simulink model "TST_APP_DD1"  (R2016b)
settings: Solver=FixedStepDiscrete  StartTime=0.0  StopTime=simTime  FixedStep=sampleTime  RelTol=1e-3
values from neighbouring files (symbols this model uses):
  testCase = 1    [initTST_APP_DD1_001.m]    (also in initTST_APP_DD1_002.m = 2)
libraries: simulink x3
settings Model: Creator=wolf072601  LastModifiedBy=wolf072601
settings DebuggingCC: SignalRangeChecking=error

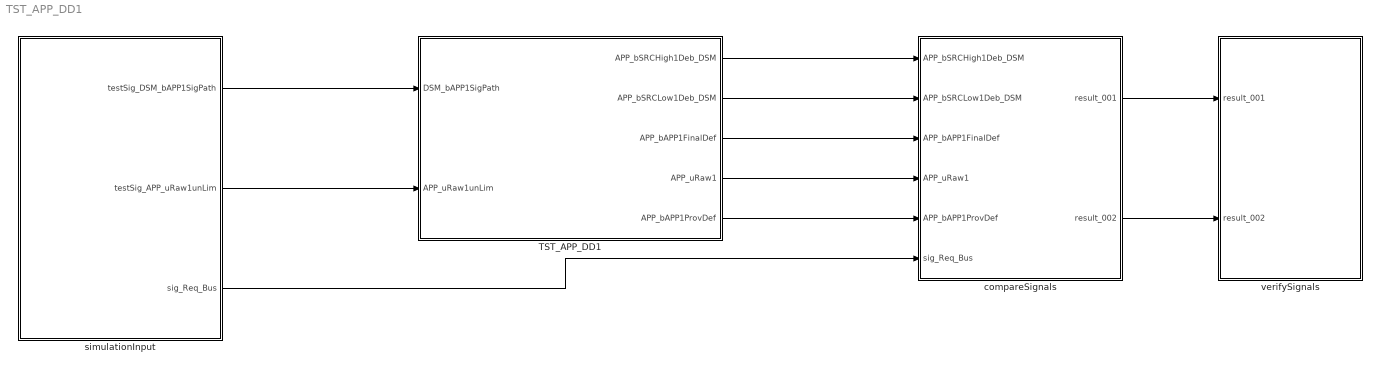
== system TST_APP_DD1 ==
  TST_APP_DD1 : Subsystem
  compareSignals : Subsystem
  simulationInput : Subsystem
  verifySignals : Subsystem
  wires:
  simulationInput/1(testSig_DSM_bAPP1SigPath) -> TST_APP_DD1/1(DSM_bAPP1SigPath)
  simulationInput/2(testSig_APP_uRaw1unLim) -> TST_APP_DD1/2(APP_uRaw1unLim)
  TST_APP_DD1/1(APP_bSRCHigh1Deb_DSM) -> compareSignals/1(APP_bSRCHigh1Deb_DSM)
  TST_APP_DD1/2(APP_bSRCLow1Deb_DSM) -> compareSignals/2(APP_bSRCLow1Deb_DSM)
  TST_APP_DD1/3(APP_bAPP1FinalDef) -> compareSignals/3(APP_bAPP1FinalDef)
  TST_APP_DD1/4(APP_uRaw1) -> compareSignals/4(APP_uRaw1)
  TST_APP_DD1/5(APP_bAPP1ProvDef) -> compareSignals/5(APP_bAPP1ProvDef)
  simulationInput/3(sig_Req_Bus) -> compareSignals/6(sig_Req_Bus)
  compareSignals/1(result_001) -> verifySignals/1(result_001)
  compareSignals/2(result_002) -> verifySignals/2(result_002)

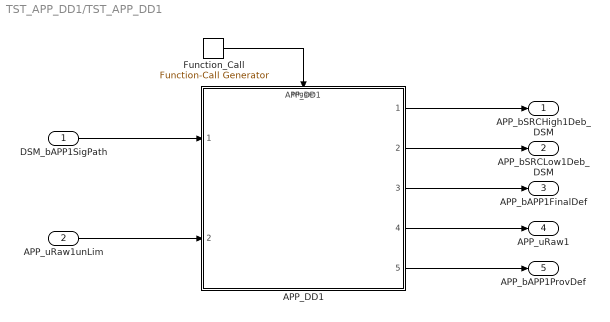
== system TST_APP_DD1/TST_APP_DD1 ==
  DSM_bAPP1SigPath : Inport
  APP_uRaw1unLim : Inport  Port=2
  APP_DD1 : ModelReference  ModelNameDialog=APP_DD1  SimulationMode=Normal  ModelReferenceVersion=1.21  TriggerPortName=function  TriggerPortTriggerType=function-call  TriggerPortStatesWhenEnabling=held
  Function_Call : simulink/Ports & Subsystems/Function-Call Generator  sample_time=sampleTime  numberOfIterations=1
  APP_bSRCHigh1Deb_DSM : Outport
  APP_bSRCLow1Deb_DSM : Outport  Port=2
  APP_bAPP1FinalDef : Outport  Port=3
  APP_uRaw1 : Outport  Port=4
  APP_bAPP1ProvDef : Outport  Port=5
  wires:
  Function_Call/1 -> APP_DD1/Trigger
  DSM_bAPP1SigPath/1 -> APP_DD1/1
  APP_uRaw1unLim/1 -> APP_DD1/2
  APP_DD1/1 -> APP_bSRCHigh1Deb_DSM/1
  APP_DD1/2 -> APP_bSRCLow1Deb_DSM/1
  APP_DD1/3 -> APP_bAPP1FinalDef/1
  APP_DD1/4 -> APP_uRaw1/1
  APP_DD1/5 -> APP_bAPP1ProvDef/1

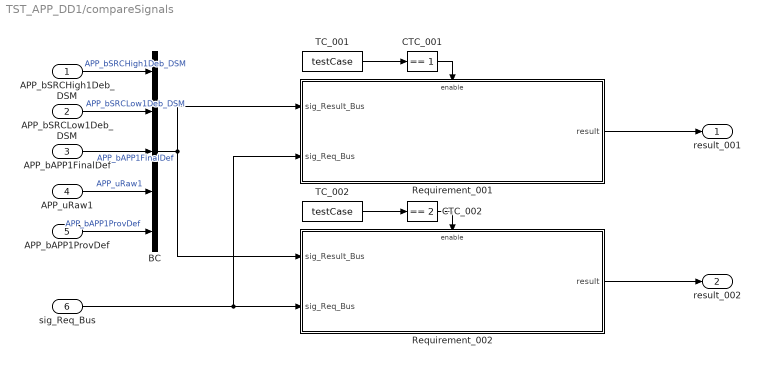
== system TST_APP_DD1/compareSignals ==
  APP_bSRCHigh1Deb_DSM : Inport
  APP_bSRCLow1Deb_DSM : Inport  Port=2
  APP_bAPP1FinalDef : Inport  Port=3
  APP_uRaw1 : Inport  Port=4
  APP_bAPP1ProvDef : Inport  Port=5
  sig_Req_Bus : Inport  Port=6
  BC : BusCreator  Inputs=5
  CTC_001 : simulink/Logic and Bit Operations/Compare To Constant  relop===  const=1  OutDataTypeStr=boolean
  CTC_002 : simulink/Logic and Bit Operations/Compare To Constant  relop===  const=2  OutDataTypeStr=boolean
  Requirement_001 : Subsystem
  Requirement_002 : Subsystem
  TC_001 : Constant  Value=testCase
  TC_002 : Constant  Value=testCase
  result_001 : Outport
  result_002 : Outport  Port=2
  wires:
  APP_bSRCHigh1Deb_DSM/1 -> BC/1  "APP_bSRCHigh1Deb_DSM"
  APP_bSRCLow1Deb_DSM/1 -> BC/2  "APP_bSRCLow1Deb_DSM"
  APP_bAPP1FinalDef/1 -> BC/3  "APP_bAPP1FinalDef"
  APP_uRaw1/1 -> BC/4  "APP_uRaw1"
  APP_bAPP1ProvDef/1 -> BC/5  "APP_bAPP1ProvDef"
  TC_001/1 -> CTC_001/1
  CTC_001/1 -> Requirement_001/Enable
  sig_Req_Bus/1 -> Requirement_002/2(sig_Req_Bus), Requirement_001/2(sig_Req_Bus)
  BC/1 -> Requirement_002/1(sig_Result_Bus), Requirement_001/1(sig_Result_Bus)
  Requirement_001/1(result) -> result_001/1
  TC_002/1 -> CTC_002/1
  CTC_002/1 -> Requirement_002/Enable
  Requirement_002/1(result) -> result_002/1

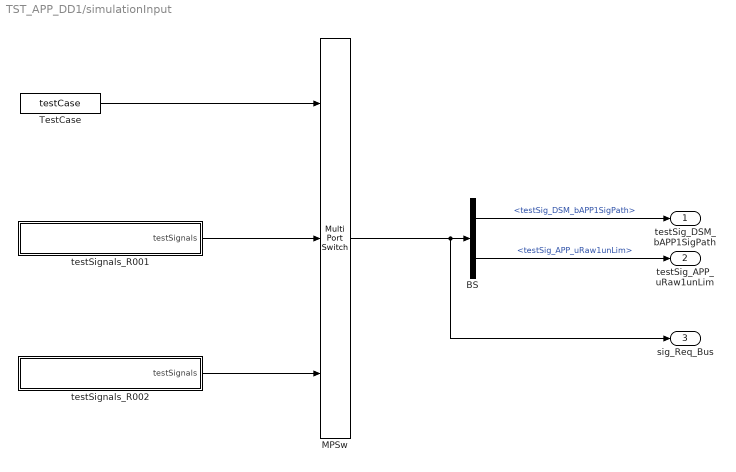
== system TST_APP_DD1/simulationInput ==
  BS : BusSelector  OutputSignals=testSig_DSM_bAPP1SigPath,testSig_APP_uRaw1unLim
  MPSw : MultiPortSwitch  Inputs=2  SaturateOnIntegerOverflow=on  InputSameDT=on
  TestCase : Constant  Value=testCase
  testSignals_R001 : Subsystem
  testSignals_R002 : Subsystem
  testSig_DSM_bAPP1SigPath : Outport
  testSig_APP_uRaw1unLim : Outport  Port=2
  sig_Req_Bus : Outport  Port=3
  wires:
  BS/1 -> testSig_DSM_bAPP1SigPath/1  "<testSig_DSM_bAPP1SigPath>"
  BS/2 -> testSig_APP_uRaw1unLim/1  "<testSig_APP_uRaw1unLim>"
  MPSw/1 -> BS/1, sig_Req_Bus/1
  TestCase/1 -> MPSw/1
  testSignals_R001/1(testSignals) -> MPSw/2
  testSignals_R002/1(testSignals) -> MPSw/3

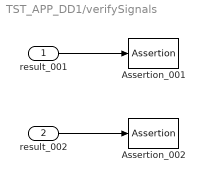
== system TST_APP_DD1/verifySignals ==
  result_001 : Inport
  result_002 : Inport  Port=2
  Assertion_001 : Assertion  Enabled=off
  Assertion_002 : Assertion
  wires:
  result_001/1 -> Assertion_001/1
  result_002/1 -> Assertion_002/1

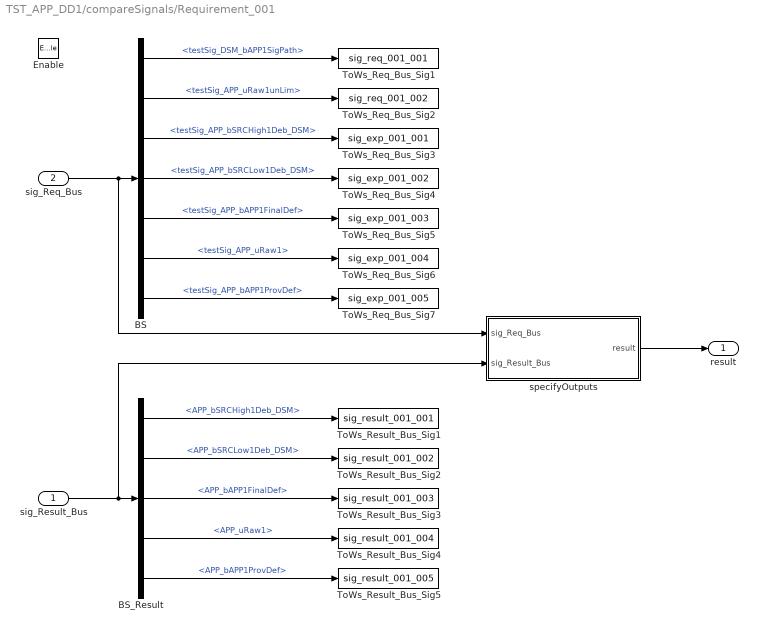
== system TST_APP_DD1/compareSignals/Requirement_001 ==
  sig_Result_Bus : Inport
  sig_Req_Bus : Inport  Port=2
  Enable : EnablePort
  BS : BusSelector  OutputSignals=testSig_DSM_bAPP1SigPath,testSig_APP_uRaw1unLim,testSig_APP_bSRCHigh1Deb_DSM,testSig_APP_bSRCLow1Deb_DSM,testSig_APP_bAPP1FinalDef,testSig_APP_uRaw1,testSig_APP_bAPP1ProvDef
  BS_Result : BusSelector  OutputSignals=APP_bSRCHigh1Deb_DSM,APP_bSRCLow1Deb_DSM,APP_bAPP1FinalDef,APP_uRaw1,APP_bAPP1ProvDef
  ToWs_Req_Bus_Sig1 : ToWorkspace  VariableName=sig_req_001_001  SaveFormat=Structure With Time
  ToWs_Req_Bus_Sig2 : ToWorkspace  VariableName=sig_req_001_002  SaveFormat=Structure With Time
  ToWs_Req_Bus_Sig3 : ToWorkspace  VariableName=sig_exp_001_001  SaveFormat=Structure With Time
  ToWs_Req_Bus_Sig4 : ToWorkspace  VariableName=sig_exp_001_002  SaveFormat=Structure With Time
  ToWs_Req_Bus_Sig5 : ToWorkspace  VariableName=sig_exp_001_003  SaveFormat=Structure With Time
  ToWs_Req_Bus_Sig6 : ToWorkspace  VariableName=sig_exp_001_004  SaveFormat=Structure With Time
  ToWs_Req_Bus_Sig7 : ToWorkspace  VariableName=sig_exp_001_005  SaveFormat=Structure With Time
  ToWs_Result_Bus_Sig1 : ToWorkspace  VariableName=sig_result_001_001  SaveFormat=Structure With Time
  ToWs_Result_Bus_Sig2 : ToWorkspace  VariableName=sig_result_001_002  SaveFormat=Structure With Time
  ToWs_Result_Bus_Sig3 : ToWorkspace  VariableName=sig_result_001_003  SaveFormat=Structure With Time
  ToWs_Result_Bus_Sig4 : ToWorkspace  VariableName=sig_result_001_004  SaveFormat=Structure With Time
  ToWs_Result_Bus_Sig5 : ToWorkspace  VariableName=sig_result_001_005  SaveFormat=Structure With Time
  specifyOutputs : Subsystem
  result : Outport
  wires:
  sig_Req_Bus/1 -> BS/1, specifyOutputs/1(sig_Req_Bus)
  BS/1 -> ToWs_Req_Bus_Sig1/1  "<testSig_DSM_bAPP1SigPath>"
  BS/2 -> ToWs_Req_Bus_Sig2/1  "<testSig_APP_uRaw1unLim>"
  BS/3 -> ToWs_Req_Bus_Sig3/1  "<testSig_APP_bSRCHigh1Deb_DSM>"
  BS/4 -> ToWs_Req_Bus_Sig4/1  "<testSig_APP_bSRCLow1Deb_DSM>"
  BS/5 -> ToWs_Req_Bus_Sig5/1  "<testSig_APP_bAPP1FinalDef>"
  BS/6 -> ToWs_Req_Bus_Sig6/1  "<testSig_APP_uRaw1>"
  BS/7 -> ToWs_Req_Bus_Sig7/1  "<testSig_APP_bAPP1ProvDef>"
  sig_Result_Bus/1 -> BS_Result/1, specifyOutputs/2(sig_Result_Bus)
  BS_Result/1 -> ToWs_Result_Bus_Sig1/1  "<APP_bSRCHigh1Deb_DSM>"
  BS_Result/2 -> ToWs_Result_Bus_Sig2/1  "<APP_bSRCLow1Deb_DSM>"
  BS_Result/3 -> ToWs_Result_Bus_Sig3/1  "<APP_bAPP1FinalDef>"
  BS_Result/4 -> ToWs_Result_Bus_Sig4/1  "<APP_uRaw1>"
  BS_Result/5 -> ToWs_Result_Bus_Sig5/1  "<APP_bAPP1ProvDef>"
  specifyOutputs/1(result) -> result/1

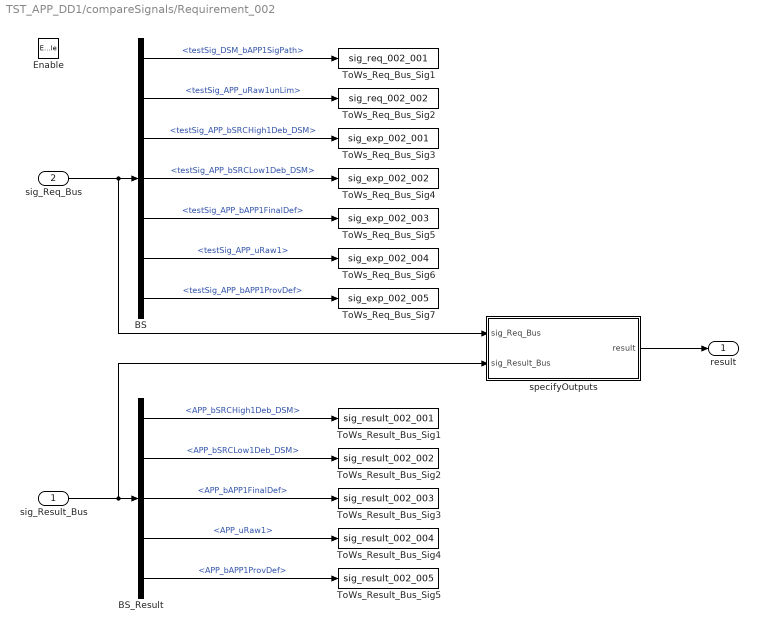
== system TST_APP_DD1/compareSignals/Requirement_002 ==
  sig_Result_Bus : Inport
  sig_Req_Bus : Inport  Port=2
  Enable : EnablePort
  BS : BusSelector  OutputSignals=testSig_DSM_bAPP1SigPath,testSig_APP_uRaw1unLim,testSig_APP_bSRCHigh1Deb_DSM,testSig_APP_bSRCLow1Deb_DSM,testSig_APP_bAPP1FinalDef,testSig_APP_uRaw1,testSig_APP_bAPP1ProvDef
  BS_Result : BusSelector  OutputSignals=APP_bSRCHigh1Deb_DSM,APP_bSRCLow1Deb_DSM,APP_bAPP1FinalDef,APP_uRaw1,APP_bAPP1ProvDef
  ToWs_Req_Bus_Sig1 : ToWorkspace  VariableName=sig_req_002_001  SaveFormat=Structure With Time
  ToWs_Req_Bus_Sig2 : ToWorkspace  VariableName=sig_req_002_002  SaveFormat=Structure With Time
  ToWs_Req_Bus_Sig3 : ToWorkspace  VariableName=sig_exp_002_001  SaveFormat=Structure With Time
  ToWs_Req_Bus_Sig4 : ToWorkspace  VariableName=sig_exp_002_002  SaveFormat=Structure With Time
  ToWs_Req_Bus_Sig5 : ToWorkspace  VariableName=sig_exp_002_003  SaveFormat=Structure With Time
  ToWs_Req_Bus_Sig6 : ToWorkspace  VariableName=sig_exp_002_004  SaveFormat=Structure With Time
  ToWs_Req_Bus_Sig7 : ToWorkspace  VariableName=sig_exp_002_005  SaveFormat=Structure With Time
  ToWs_Result_Bus_Sig1 : ToWorkspace  VariableName=sig_result_002_001  SaveFormat=Structure With Time
  ToWs_Result_Bus_Sig2 : ToWorkspace  VariableName=sig_result_002_002  SaveFormat=Structure With Time
  ToWs_Result_Bus_Sig3 : ToWorkspace  VariableName=sig_result_002_003  SaveFormat=Structure With Time
  ToWs_Result_Bus_Sig4 : ToWorkspace  VariableName=sig_result_002_004  SaveFormat=Structure With Time
  ToWs_Result_Bus_Sig5 : ToWorkspace  VariableName=sig_result_002_005  SaveFormat=Structure With Time
  specifyOutputs : Subsystem
  result : Outport
  wires:
  sig_Req_Bus/1 -> BS/1, specifyOutputs/1(sig_Req_Bus)
  BS/1 -> ToWs_Req_Bus_Sig1/1  "<testSig_DSM_bAPP1SigPath>"
  BS/2 -> ToWs_Req_Bus_Sig2/1  "<testSig_APP_uRaw1unLim>"
  BS/3 -> ToWs_Req_Bus_Sig3/1  "<testSig_APP_bSRCHigh1Deb_DSM>"
  BS/4 -> ToWs_Req_Bus_Sig4/1  "<testSig_APP_bSRCLow1Deb_DSM>"
  BS/5 -> ToWs_Req_Bus_Sig5/1  "<testSig_APP_bAPP1FinalDef>"
  BS/6 -> ToWs_Req_Bus_Sig6/1  "<testSig_APP_uRaw1>"
  BS/7 -> ToWs_Req_Bus_Sig7/1  "<testSig_APP_bAPP1ProvDef>"
  sig_Result_Bus/1 -> BS_Result/1, specifyOutputs/2(sig_Result_Bus)
  BS_Result/1 -> ToWs_Result_Bus_Sig1/1  "<APP_bSRCHigh1Deb_DSM>"
  BS_Result/2 -> ToWs_Result_Bus_Sig2/1  "<APP_bSRCLow1Deb_DSM>"
  BS_Result/3 -> ToWs_Result_Bus_Sig3/1  "<APP_bAPP1FinalDef>"
  BS_Result/4 -> ToWs_Result_Bus_Sig4/1  "<APP_uRaw1>"
  BS_Result/5 -> ToWs_Result_Bus_Sig5/1  "<APP_bAPP1ProvDef>"
  specifyOutputs/1(result) -> result/1

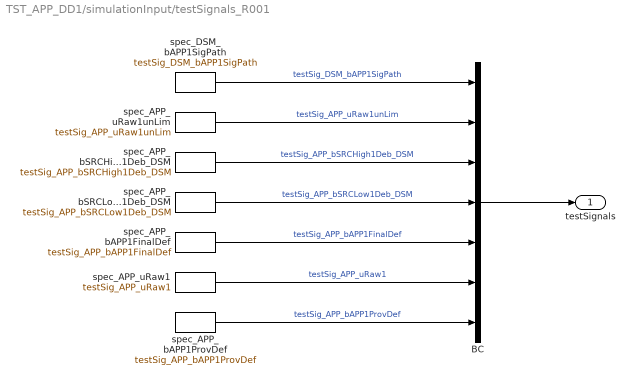
== system TST_APP_DD1/simulationInput/testSignals_R001 ==
  BC : BusCreator  Inputs=7
  spec_APP_bAPP1FinalDef : FromWorkspace  VariableName=testSig_APP_bAPP1FinalDef  Interpolate=off  OutputAfterFinalValue=Holding final value
  spec_APP_bAPP1ProvDef : FromWorkspace  VariableName=testSig_APP_bAPP1ProvDef  Interpolate=off  OutputAfterFinalValue=Holding final value
  spec_APP_bSRCHigh1Deb_DSM : FromWorkspace  VariableName=testSig_APP_bSRCHigh1Deb_DSM  Interpolate=off  OutputAfterFinalValue=Holding final value
  spec_APP_bSRCLow1Deb_DSM : FromWorkspace  VariableName=testSig_APP_bSRCLow1Deb_DSM  Interpolate=off  OutputAfterFinalValue=Holding final value
  spec_APP_uRaw1 : FromWorkspace  VariableName=testSig_APP_uRaw1  Interpolate=off  OutputAfterFinalValue=Holding final value
  spec_APP_uRaw1unLim : FromWorkspace  VariableName=testSig_APP_uRaw1unLim  Interpolate=off  OutputAfterFinalValue=Holding final value
  spec_DSM_bAPP1SigPath : FromWorkspace  VariableName=testSig_DSM_bAPP1SigPath  Interpolate=off  OutputAfterFinalValue=Holding final value
  testSignals : Outport
  wires:
  BC/1 -> testSignals/1
  spec_DSM_bAPP1SigPath/1 -> BC/1  "testSig_DSM_bAPP1SigPath"
  spec_APP_uRaw1unLim/1 -> BC/2  "testSig_APP_uRaw1unLim"
  spec_APP_bSRCHigh1Deb_DSM/1 -> BC/3  "testSig_APP_bSRCHigh1Deb_DSM"
  spec_APP_bSRCLow1Deb_DSM/1 -> BC/4  "testSig_APP_bSRCLow1Deb_DSM"
  spec_APP_bAPP1FinalDef/1 -> BC/5  "testSig_APP_bAPP1FinalDef"
  spec_APP_uRaw1/1 -> BC/6  "testSig_APP_uRaw1"
  spec_APP_bAPP1ProvDef/1 -> BC/7  "testSig_APP_bAPP1ProvDef"

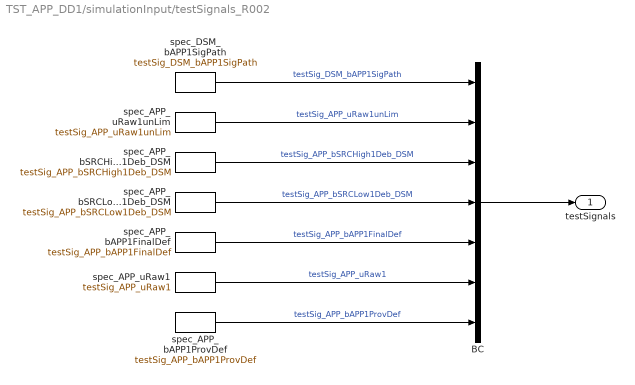
== system TST_APP_DD1/simulationInput/testSignals_R002 ==
  BC : BusCreator  Inputs=7
  spec_APP_bAPP1FinalDef : FromWorkspace  VariableName=testSig_APP_bAPP1FinalDef  Interpolate=off  OutputAfterFinalValue=Holding final value
  spec_APP_bAPP1ProvDef : FromWorkspace  VariableName=testSig_APP_bAPP1ProvDef  Interpolate=off  OutputAfterFinalValue=Holding final value
  spec_APP_bSRCHigh1Deb_DSM : FromWorkspace  VariableName=testSig_APP_bSRCHigh1Deb_DSM  Interpolate=off  OutputAfterFinalValue=Holding final value
  spec_APP_bSRCLow1Deb_DSM : FromWorkspace  VariableName=testSig_APP_bSRCLow1Deb_DSM  Interpolate=off  OutputAfterFinalValue=Holding final value
  spec_APP_uRaw1 : FromWorkspace  VariableName=testSig_APP_uRaw1  Interpolate=off  OutputAfterFinalValue=Holding final value
  spec_APP_uRaw1unLim : FromWorkspace  VariableName=testSig_APP_uRaw1unLim  Interpolate=off  OutputAfterFinalValue=Holding final value
  spec_DSM_bAPP1SigPath : FromWorkspace  VariableName=testSig_DSM_bAPP1SigPath  Interpolate=off  OutputAfterFinalValue=Holding final value
  testSignals : Outport
  wires:
  BC/1 -> testSignals/1
  spec_DSM_bAPP1SigPath/1 -> BC/1  "testSig_DSM_bAPP1SigPath"
  spec_APP_uRaw1unLim/1 -> BC/2  "testSig_APP_uRaw1unLim"
  spec_APP_bSRCHigh1Deb_DSM/1 -> BC/3  "testSig_APP_bSRCHigh1Deb_DSM"
  spec_APP_bSRCLow1Deb_DSM/1 -> BC/4  "testSig_APP_bSRCLow1Deb_DSM"
  spec_APP_bAPP1FinalDef/1 -> BC/5  "testSig_APP_bAPP1FinalDef"
  spec_APP_uRaw1/1 -> BC/6  "testSig_APP_uRaw1"
  spec_APP_bAPP1ProvDef/1 -> BC/7  "testSig_APP_bAPP1ProvDef"

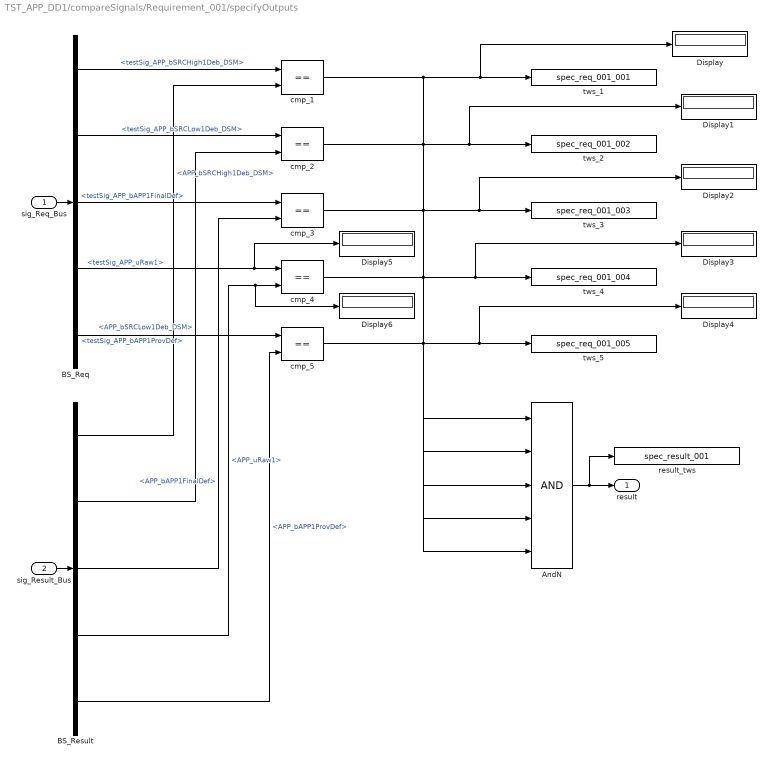
== system TST_APP_DD1/compareSignals/Requirement_001/specifyOutputs ==
  sig_Req_Bus : Inport
  sig_Result_Bus : Inport  Port=2
  AndN : Logic  Inputs=5
  BS_Req : BusSelector  OutputSignals=testSig_APP_bSRCHigh1Deb_DSM,testSig_APP_bSRCLow1Deb_DSM,testSig_APP_bAPP1FinalDef,testSig_APP_uRaw1,testSig_APP_bAPP1ProvDef
  BS_Result : BusSelector  OutputSignals=APP_bSRCHigh1Deb_DSM,APP_bSRCLow1Deb_DSM,APP_bAPP1FinalDef,APP_uRaw1,APP_bAPP1ProvDef
  Display{,1..6} (7 alike) : Display
  cmp_{1..5} (5 alike) : RelationalOperator  Operator===  RndMeth=Nearest  InputSameDT=on
  result_tws : ToWorkspace  VariableName=spec_result_001
  tws_1 : ToWorkspace  VariableName=spec_req_001_001
  tws_2 : ToWorkspace  VariableName=spec_req_001_002
  tws_3 : ToWorkspace  VariableName=spec_req_001_003
  tws_4 : ToWorkspace  VariableName=spec_req_001_004
  tws_5 : ToWorkspace  VariableName=spec_req_001_005
  result : Outport
  wires:
  sig_Req_Bus/1 -> BS_Req/1
  sig_Result_Bus/1 -> BS_Result/1
  AndN/1 -> result/1, result_tws/1
  BS_Req/1 -> cmp_1/1  "<testSig_APP_bSRCHigh1Deb_DSM>"
  BS_Result/1 -> cmp_1/2  "<APP_bSRCHigh1Deb_DSM>"
  cmp_1/1 -> Display/1, tws_1/1, AndN/1
  BS_Req/2 -> cmp_2/1  "<testSig_APP_bSRCLow1Deb_DSM>"
  BS_Result/2 -> cmp_2/2  "<APP_bSRCLow1Deb_DSM>"
  cmp_2/1 -> Display1/1, tws_2/1, AndN/2
  BS_Req/3 -> cmp_3/1  "<testSig_APP_bAPP1FinalDef>"
  BS_Result/3 -> cmp_3/2  "<APP_bAPP1FinalDef>"
  BS_Req/4 -> Display5/1, cmp_4/1  "<testSig_APP_uRaw1>"
  BS_Result/4 -> Display6/1, cmp_4/2  "<APP_uRaw1>"
  cmp_4/1 -> Display3/1, tws_4/1, AndN/4
  BS_Req/5 -> cmp_5/1  "<testSig_APP_bAPP1ProvDef>"
  BS_Result/5 -> cmp_5/2  "<APP_bAPP1ProvDef>"
  cmp_5/1 -> Display4/1, tws_5/1, AndN/5
  cmp_3/1 -> Display2/1, tws_3/1, AndN/3

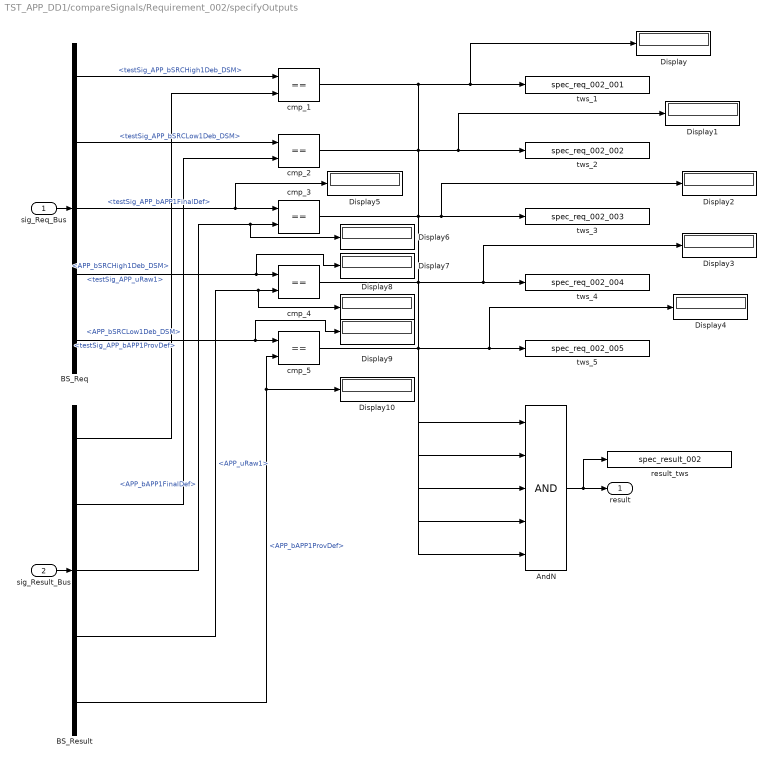
== system TST_APP_DD1/compareSignals/Requirement_002/specifyOutputs ==
  sig_Req_Bus : Inport
  sig_Result_Bus : Inport  Port=2
  AndN : Logic  Inputs=5
  BS_Req : BusSelector  OutputSignals=testSig_APP_bSRCHigh1Deb_DSM,testSig_APP_bSRCLow1Deb_DSM,testSig_APP_bAPP1FinalDef,testSig_APP_uRaw1,testSig_APP_bAPP1ProvDef
  BS_Result : BusSelector  OutputSignals=APP_bSRCHigh1Deb_DSM,APP_bSRCLow1Deb_DSM,APP_bAPP1FinalDef,APP_uRaw1,APP_bAPP1ProvDef
  Display{,1..10} (11 alike) : Display
  cmp_{1..5} (5 alike) : RelationalOperator  Operator===  RndMeth=Nearest  InputSameDT=on
  result_tws : ToWorkspace  VariableName=spec_result_002
  tws_1 : ToWorkspace  VariableName=spec_req_002_001
  tws_2 : ToWorkspace  VariableName=spec_req_002_002
  tws_3 : ToWorkspace  VariableName=spec_req_002_003
  tws_4 : ToWorkspace  VariableName=spec_req_002_004
  tws_5 : ToWorkspace  VariableName=spec_req_002_005
  result : Outport
  wires:
  sig_Req_Bus/1 -> BS_Req/1
  sig_Result_Bus/1 -> BS_Result/1
  AndN/1 -> result/1, result_tws/1
  BS_Req/1 -> cmp_1/1  "<testSig_APP_bSRCHigh1Deb_DSM>"
  BS_Result/1 -> cmp_1/2  "<APP_bSRCHigh1Deb_DSM>"
  cmp_1/1 -> Display/1, tws_1/1, AndN/1
  BS_Req/2 -> cmp_2/1  "<testSig_APP_bSRCLow1Deb_DSM>"
  BS_Result/2 -> cmp_2/2  "<APP_bSRCLow1Deb_DSM>"
  cmp_2/1 -> Display1/1, tws_2/1, AndN/2
  BS_Req/3 -> Display5/1, cmp_3/1  "<testSig_APP_bAPP1FinalDef>"
  BS_Result/3 -> Display6/1, cmp_3/2  "<APP_bAPP1FinalDef>"
  cmp_3/1 -> Display2/1, tws_3/1, AndN/3
  BS_Req/4 -> Display7/1, cmp_4/1  "<testSig_APP_uRaw1>"
  BS_Result/4 -> Display8/1, cmp_4/2  "<APP_uRaw1>"
  cmp_4/1 -> Display3/1, tws_4/1, AndN/4
  BS_Req/5 -> Display9/1, cmp_5/1  "<testSig_APP_bAPP1ProvDef>"
  BS_Result/5 -> Display10/1, cmp_5/2  "<APP_bAPP1ProvDef>"
  cmp_5/1 -> Display4/1, tws_5/1, AndN/5
